simulink model "Exo_Origianl"  (R2023b)
settings: Solver=ode5  StartTime=0.0  StopTime=inf  FixedStep=dt  RelTol=1e-3  EnableMultiTasking=on
values from neighbouring files (symbols this model uses):
  A_0_a = 4.011    [Operator.m]
  A_0_h = 40.69    [Operator.m]
  A_0_k = 25.7    [Operator.m]
  A_1_a = 5.292    [Operator.m]
  A_1_h = 23.22    [Operator.m]
  A_1_k = -3.827    [Operator.m]
  A_2_a = -8.582    [Operator.m]
  A_2_h = -4.487    [Operator.m]
  A_2_k = -8.543    [Operator.m]
  A_3_a = -0.4755    [Operator.m]
  A_3_h = 0.3995    [Operator.m]
  A_3_k = 1.913    [Operator.m]
  A_4_a = 1.688    [Operator.m]
  A_4_k = 1.087    [Operator.m]
  A_5_a = -0.03504    [Operator.m]
  A_5_k = 2.054    [Operator.m]
  A_6_a = 1.298    [Operator.m]
  A_6_k = -0.3061    [Operator.m]
  amplitude = 0.8    [Operator.m]
  ankleStrategyInterval = 1.5    [Operator.m]
  B_1_a = 3.613    [Operator.m]
  B_1_h = -8.65    [Operator.m]
  B_1_k = -19.28    [Operator.m]
  B_2_a = -5.954    [Operator.m]
  B_2_h = 3.338    [Operator.m]
  B_2_k = 17.93    [Operator.m]
  B_3_a = 5.918    [Operator.m]
  B_3_h = 1.389    [Operator.m]
  B_3_k = 3.772    [Operator.m]
  B_4_a = -2.118    [Operator.m]
  B_4_k = 1.504    [Operator.m]
  B_5_a = 1.023    [Operator.m]
  B_5_k = 0.5838    [Operator.m]
  B_6_a = -0.7245    [Operator.m]
  B_6_k = -0.8958    [Operator.m]
  DCM_filter = 1 - dt/(dt+RC)    (= 0.926612305411)    [Operator.m]
  dt = 0.01    [Operator.m]
  frequency = 1.2    [Operator.m]
  gamma = fzero(eqn, 0.1)    [Operator.m]
  hipOffset = -17    [Operator.m]
  K_high = 0.5    [Operator.m]
  K_low = 0.5    [Operator.m]
  KD = 0.39    [Operator.m]
  Kp = 10    [Operator.m]
  l3 = userHeight*0.232    (= 15.776)    [Operator.m]
  l4 = userHeight*0.247    (= 16.796)    [Operator.m]
  l_c2 = ((0.29*34.66+0.63*6.07)/(6.07+34.66))/(0.52+0.19)*l2    (= 15.0425832454)    [Operator.m]
  l_c3 = 0.17/0.40*l3    (= 6.7048)    [Operator.m]
  l_c4 = ((0.19*3.52+0.43*1.05)/(3.52+1.05))/0.43*l4    (= 9.57536959951)    [Operator.m]
  l_foot = 11.25    [Operator.m]
  m2 = m2 + 2.2048*7.591    (= 119.8566368)    [Operator.m]
  m3 = m3 + 2.2048*1.715    (= 19.781232)    [Operator.m]
  m4 = userWeight*(0.0459+0.0169)    (= 10.048)    [Operator.m]
  m_Exo = 2.2048*1.647    (= 3.6313056)    [Operator.m]
  m_f = userWeight*0.0169    (= 2.704)    [Operator.m]
  maxTorque = 35    [Operator.m]
  P_t_ZMP_gain_Ankle = 0    [Operator.m]
  P_t_ZMP_gain_Hip = 0    [Operator.m]
  Phase_Left = 2+pi    (= 5.14159265359)    [Operator.m]
  Phase_Right = 2    [Operator.m]
  ramp = 2    [Operator.m]
  Strategy_filter = DCM_filter    (= 0.926612305411)    [Operator.m]
  strategySaturation = 10    [Operator.m]
  userHeight = 68    [Operator.m]
  userWeight = 160    [Operator.m]
undefined symbols (not defined in the file or in its folder): CAN_Device, DCMErrorPenalty, PEAK, Phase_Left_Knee_0, System, totalPowerPenalty
libraries: sldrtlib x35, simulink x16, rllib x1
(part 1 of 4)
settings Model: SimulationMode=external  ExtModeTrigDuration=60001  Creator=517541  LastModifiedBy=tschmidt
settings SolverCC: AlgebraicLoopSolver=TrustRegion
settings DataIOCC: ReturnWorkspaceOutputs=off
settings DebuggingCC: SolverPrmCheckMsg=warning  UnconnectedInputMsg=warning  UnconnectedOutputMsg=warning  UnconnectedLineMsg=warning  PregeneratedLibrarySubsystemCodeDiagnostic=none  SFUnexpectedBacktrackingDiag=warning  SFNoUnconditionalDefaultTransitionDiag=warning  SFExecutionAtInitializationDiag=none  ArithmeticOperatorsInVariantConditions=warning
settings HardwareCC: ProdBitPerLong=64  ProdHWDeviceType=Intel->x86-64 (Linux 64)
settings ModelReferenceCC: EnableRefExpFcnMdlSchedulingChecks=on  PropagateSignalLabelsOutOfModel=off
settings SFSimCC: SimUseLocalCustomCode=off  CustomCodeUndefinedFunction=UseInterfaceOnly
settings RTWCC: Description=Simulink Desktop Real-Time  SystemTargetFile=sldrt.tlc  TemplateMakefile=sldrt.tmf  RTWUseLocalCustomCode=off  RTWCompilerOptimization=on  DLArmComputeVersion=19.05
settings CodeAppCC: MaxIdLength=95  StateflowObjectComments=on
settings SimulinkDesktopRealTimeCC: TargetLibSuffix=_sldrt.a  TargetPreCompLibLocation=C:\Program Files\MATLAB\R2023b\toolbox\sldrt\lib\win64

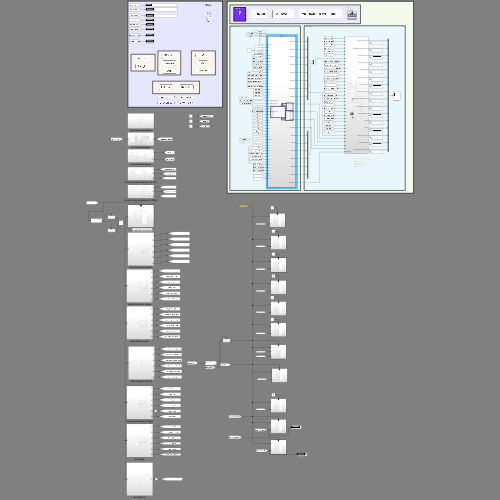
[thumbnail: Simulink's stored preview of the top-level diagram]
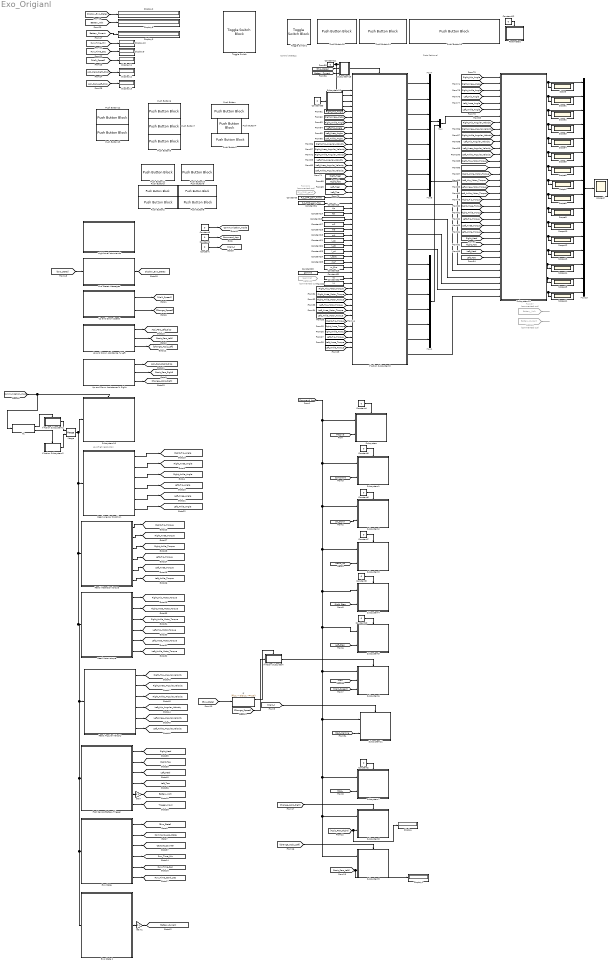
== system Exo_Origianl ==
  note: Control Strategy
  note: Data Retrieval
  note: Low/High resolution
  Constant{,1..2,4..12,33} (13 alike) : Constant  Value=0
  Constant13 : Constant  Value=Kp
  Constant14 : Constant  Value=KD
  Constant15 : Constant  Value=ankleStrategyInterval
  Constant17 : Constant  Value=m2
  Constant18 : Constant  Value=m3
  Constant19 : Constant  Value=m4
  Constant21 : Constant  Value=l_c2
  Constant22 : Constant  Value=l_c3
  Constant23 : Constant  Value=l_c4
  Constant24 : Constant  Value=l_foot
  Constant25 : Constant  Value=m_f
  Constant26 : Constant  Value=m_Exo
  Constant28 : Constant  Value=gamma
  Constant3 : Constant  Value=P_t_ZMP_gain_Ankle
  Constant31 : Constant  Value=l3
  Constant32 : Constant  Value=l4
  Constant34 : Constant  Value=P_t_ZMP_gain_Hip
  Display{,1..3,8..13} (10 alike) : Display
  Exo State : Subsystem
  Exo State 2 : Subsystem
  Exo States Messages : Subsystem
  Foot Sensor/Battery/Trigger : Subsystem
  From101 : From  Commented=on  GotoTag=P_t_ZMP_gain
  From102 : From  Commented=on  GotoTag=gamma
  From37 : From  Commented=on  GotoTag=Battery_Volt  TagVisibility=global
  From38 : From  Commented=on  GotoTag=Battery_Current  TagVisibility=global
  Gain : Gain  Gain=0.1
  Gain1 : Gain  Gain=0.1
  High-level commands : Subsystem
  If : If  IfExpression=(u1 > 0)&(u1 <= 10)
  If Action Subsystem : Subsystem  TreatAsAtomicUnit=on
  If Action Subsystem1 : Subsystem  TreatAsAtomicUnit=on
  If Action Subsystem2 : Subsystem  TreatAsAtomicUnit=on
  If Action Subsystem3 : Subsystem  TreatAsAtomicUnit=on
  If1 : If
  Merge : Merge
  Mux : Mux  Inputs=2
  Mux1 : Mux  Inputs=6
  Mux13 : Mux  Inputs=16
  Mux5 : Mux  Inputs=2
  Mux7 : Mux  Inputs=6
  Parameters : Subsystem
  Push Button : PushButtonBlock  ButtonText=Up Vel  OffValue=0.000000
  Push Button1 : PushButtonBlock  ButtonText=Down Vel
  Push Button10 : PushButtonBlock  ButtonText=Right_Step  OffValue=0.000000
  Push Button11 : PushButtonBlock  ButtonText=Left_Step  OffValue=0.000000
  Push Button12 : PushButtonBlock  ButtonText=Sit_Down  OffValue=0.000000
  Push Button13 : PushButtonBlock  ButtonText=Stand_Up  OffValue=0.000000
  Push Button14 : PushButtonBlock  ButtonText=Walk/Stop  ButtonType=Latch  OffValue=0.000000
  Push Button15 : PushButtonBlock  ButtonText=Acknowledge Parameters  OffValue=0.000000
  Push Button16 : PushButtonBlock  ButtonText=Activate  ButtonType=Latch  OffValue=0.000000
  Push Button2 : PushButtonBlock  ButtonText=Down Left %  OffValue=0.000000
  Push Button3 : PushButtonBlock  ButtonText=Up Left %  OffValue=0.000000
  Push Button4 : PushButtonBlock  ButtonText=Walk  OffValue=0.000000
  Push Button5 : PushButtonBlock  ButtonText=Stop  OffValue=0.000000
  Push Button6 : PushButtonBlock  ButtonText=Release  OffValue=0.000000
  Push Button7 : PushButtonBlock  ButtonText=Transparent  OffValue=0.000000
  Push Button8 : PushButtonBlock  ButtonText=Down Right %  OffValue=0.000000
  Push Button9 : PushButtonBlock  ButtonText=Up Right %  OffValue=0.000000
  Read Angular Possition : Subsystem
  Read Angular Velocity : Subsystem
  Read Interaction torque : Subsystem
  Read Motor torque : Subsystem
  Scope{,1..15} (16 alike) : Scope
  Subsystem : Subsystem
  Subsystem1 : Subsystem
  Subsystem10 : Subsystem
  Subsystem11 : Subsystem
  Subsystem12 : Subsystem
  Subsystem13 : Subsystem
  Subsystem15 : Subsystem
  Subsystem2 : Subsystem
  Subsystem3 : Subsystem
  Subsystem4 : Subsystem
  Subsystem5 : Subsystem
  Subsystem6 : Subsystem
  Subsystem7 : Subsystem
  Subsystem8 : Subsystem
  Subsystem9 : Subsystem
  Toggle Switch : ToggleSwitchBlock
      settings: Values={{'CAN', 'Bluetooth'}, [0 1]}
  Toggle Switch1 : ToggleSwitchBlock  LabelPosition=Hide
      settings: Values={{'Low resolution', 'High resolution'}, [1 0]}
  Up and Down Assistance % Left : Subsystem
  Up and Down Assistance % Right : Subsystem
  Up and Down Speed : Subsystem
  scopeAll : Scope
  tag scope: Assi_Perc_Left_Disp=global, Assi_Perc_Right_Disp=global, Battery_Current=global, Battery_Volt=global, Capture_Counter=global, Change_Assis_Right=global, Command_App=global, Command_App_State=global, Communication_mode=global, Display_Exo_States=global, Left_Ankle_Angle=global, Left_Ankle_Angular_Velocity=global, Left_Ankle_Motor_Torque=global, Left_Ankle_Torque=global, Left_Heel=global, Left_Hip_Angle=global, Left_Hip_Angular_Velocity=global, Left_Hip_Motor_Torque=global, Left_Hip_Torque=global, Left_Knee_Angle=global, Left_Knee_Angular_Velocity=global, Left_Knee_Motor_Torque=global, Left_Knee_Torque=global, Left_Toe=global, Right_Ankle_Angle=global, Right_Ankle_Angular_Velocity=global, Right_Ankle_Motor_Torque=global, Right_Ankle_Torque=global, Right_Heel=global, Right_Hip_Angle=global, Right_Hip_Angular_Velocity=global, Right_Hip_Motor_Torque=global, Right_Hip_Torque=global, Right_Knee_Angle=global, Right_Knee_Angular_Velocity=global, Right_Knee_Motor_Torque=global, Right_Knee_Torque=global, Right_Toe=global, Run_Time_Centi_Sec=global, Run_Time_Min=global, Run_Time_Sec=global, Trigger_Input=global
  wires:
  Constant1/1 -> [Command_App]
  [Compliant] -> Subsystem1/2(In2)
  Up and Down Speed/1(Out1) -> [Walk_Speed]
  [Sit_Down] -> Subsystem2/2(In2)
  [Stand_Up] -> Subsystem3/2(In2)
  [Right_Step] -> Subsystem4/2(In2)
  [Left_Step] -> Subsystem5/2(In2)
  [Passive] -> Subsystem/2(In2)
  Constant/1 -> [Walk_]
  Constant4/1 -> Subsystem/Trigger
  Constant10/1 -> Subsystem5/Trigger
  Constant8/1 -> Subsystem4/Trigger
  Constant7/1 -> Subsystem3/Trigger
  Constant6/1 -> Subsystem2/Trigger
  Constant5/1 -> Subsystem1/Trigger
  Up and Down Assistance % Right/3(Out3) -> [Change_Assis_Right]
  Up and Down Assistance % Right/2(Out2) -> [Assis_Perc_Right]
  Up and Down Assistance % Right/1(Out1) -> [Assi_Perc_Right_Disp]
  [Exo_State] -> Exo States Messages/1(In1)
  Exo States Messages/1(Out1) -> [Display_Exo_States]
  [Assi_Perc_Right_Disp] -> Display12/1
  [Assi_Perc_Left_Disp] -> Display13/1
  [Run_Time_Min] -> Display10/1
  [Display_Exo_States] -> Display2/1
  [Run_Time_Sec] -> Display9/1
  [Walk_Speed] -> Display11/1
  [Battery_Volt] -> Display8/1
  Read Interaction torque/4(Out4) -> [Left_Hip_Torque]
  Read Interaction torque/2(Out2) -> [Right_Knee_Torque]
  Read Interaction torque/3(Out3) -> [Right_Ankle_Torque]
  Read Interaction torque/6(Out6) -> [Left_Ankle_Torque]
  Read Interaction torque/1(Out1) -> [Right_Hip_Torque]
  Read Interaction torque/5(Out5) -> [Left_Knee_Torque]
  Read Motor torque/2(Out2) -> [Right_Knee_Motor_Torque]
  Read Motor torque/5(Out5) -> [Left_Knee_Motor_Torque]
  Read Motor torque/3(Out3) -> [Right_Ankle_Motor_Torque]
  Read Motor torque/1(Out1) -> [Right_Hip_Motor_Torque]
  Read Motor torque/6(Out6) -> [Left_Ankle_Motor_Torque]
  Read Motor torque/4(Out4) -> [Left_Hip_Motor_Torque]
  Foot Sensor/Battery/Trigger/4(Out4) -> [Left_Toe]
  Foot Sensor/Battery/Trigger/6(Out6) -> [Trigger_Input]
  Foot Sensor/Battery/Trigger/2(Out2) -> [Right_Toe]
  Foot Sensor/Battery/Trigger/1(Out1) -> [Right_Heel]
  Foot Sensor/Battery/Trigger/3(Out3) -> [Left_Heel]
  Exo State/4(Out4) -> [Run_Time_Min]
  Exo State/1(Out1) -> [Exo_State]
  Exo State/2(Out2) -> [Command_App_State]
  Exo State/5(Out5) -> [Run_Time_Sec]
  Exo State/6(Out6) -> [Run_Time_Centi_Sec]
  Exo State/3(Out3) -> [Capture_Counter]
  Gain/1 -> [Battery_Volt]
  Foot Sensor/Battery/Trigger/5(Out5) -> Gain/1
  Up and Down Assistance % Left/1(Out1) -> [Assi_Perc_Left_Disp]
  Up and Down Assistance % Left/2(Out2) -> [Assis_Perc_Left]
  Up and Down Assistance % Left/3(Out3) -> [Change_Assis_Left]
  [Start_Walking] -> Subsystem11/2(In2)
  [Assis_Perc_Right] -> Display/1, Subsystem8/2(In2)
  If/1 -> If Action Subsystem/Action
  [Assis_Perc_Left] -> Display1/1, Subsystem9/2(In2)
  [Stop_] -> Subsystem7/2(In2)
  [Change_Assis_Left] -> Subsystem9/Trigger
  [Change_Speed] -> If Action Subsystem/1(In1)
  [Walk_] -> Subsystem11/Trigger
  [Change_Assis_Right] -> Subsystem8/Trigger
  [Command_App] -> Subsystem/1(In1), Subsystem1/1(In1), Subsystem2/1(In1), Subsystem3/1(In1), Subsystem4/1(In1), Subsystem11/1(In1), Subsystem9/1(In1), Subsystem8/1(In1), Subsystem7/1(In1), Subsystem6/1(In1), Subsystem5/1(In1)
  [Walk] -> Subsystem6/2(In2)
  If Action Subsystem/1(Out1) -> Subsystem6/Trigger
  Constant2/1 -> Subsystem7/Trigger
  [Walk_Speed] -> Subsystem6/3(In3)
  [Exo_State] -> If/1
  Up and Down Speed/2(Out2) -> [Change_Speed]
  [Communication_mode] -> If1/1, Subsystem10/Trigger
  Constant9/1 -> [Communication_mode]
  Read Angular Possition/1(Out1) -> [Right_Hip_Angle]
  Read Angular Possition/2(Out2) -> [Right_Knee_Angle]
  Read Angular Possition/3(Out3) -> [Right_Ankle_Angle]
  Read Angular Possition/4(Out4) -> [Left_Hip_Angle]
  Read Angular Possition/5(Out5) -> [Left_Knee_Angle]
  Read Angular Possition/6(Out6) -> [Left_Ankle_Angle]
  If1/1 -> If Action Subsystem1/Action
  If Action Subsystem1/1(Out1) -> Merge/1
  If1/2 -> If Action Subsystem2/Action
  If Action Subsystem2/1(Out1) -> Merge/2
  Merge/1 -> Read Angular Velocity/1(Input), Exo State 2/1(Input), Exo State/1(Input), Foot Sensor/Battery/Trigger/1(Input), Read Motor torque/1(Input), Read Interaction torque/1(Input), Read Angular Possition/1(Input), Subsystem10/1(In1)
  Exo State 2/1(Out1) -> Gain1/1
  Gain1/1 -> [Battery_Current]
  [Battery_Current] -> Display3/1
  Read Angular Velocity/4(Out4) -> [Left_Hip_Angular_Velocity]
  Read Angular Velocity/6(Out6) -> [Left_Ankle_Angular_Velocity]
  Read Angular Velocity/3(Out3) -> [Right_Ankle_Angular_Velocity]
  Read Angular Velocity/5(Out5) -> [Left_Knee_Angular_Velocity]
  Read Angular Velocity/2(Out2) -> [Right_Knee_Angular_Velocity]
  Read Angular Velocity/1(Out1) -> [Right_Hip_Angular_Velocity]
  Constant11/1 -> If Action Subsystem3/1(Trigger), Subsystem15/1(Input)
  [Right_Hip_Angle] -> If Action Subsystem3/5(RHAA)
  [Right_Knee_Angle] -> If Action Subsystem3/6(RKAA)
  [Right_Ankle_Angle] -> If Action Subsystem3/7(RAAA)
  [Left_Hip_Angle] -> If Action Subsystem3/8(LHAA)
  [Left_Knee_Angle] -> If Action Subsystem3/9(LKAA)
  [Left_Ankle_Angle] -> If Action Subsystem3/10(LAAA)
  [Right_Heel] -> If Action Subsystem3/17(RHP)
  [Right_Toe] -> If Action Subsystem3/18(RTP)
  [Left_Heel] -> If Action Subsystem3/19(LHP)
  [Left_Toe] -> If Action Subsystem3/20(LTP)
  [Left_Ankle_Angular_Velocity] -> If Action Subsystem3/16(Input5)
  [Right_Ankle_Angular_Velocity] -> If Action Subsystem3/13(Input4)
  Subsystem15/1(Trigger) -> If Action Subsystem3/Action
  [Right_Hip_Angular_Velocity] -> If Action Subsystem3/11(Input2)
  [Left_Hip_Angular_Velocity] -> If Action Subsystem3/14(Input14)
  [Left_Knee_Angular_Velocity] -> If Action Subsystem3/15(Input15)
  [Right_Knee_Angular_Velocity] -> If Action Subsystem3/12(Input3)
  Constant12/1 -> Parameters/Trigger
  Subsystem12/1(amplitude) -> If Action Subsystem3/2(Input6)
  Subsystem12/2(frequency) -> If Action Subsystem3/3(Input7)
  Subsystem12/3(hipOffset) -> If Action Subsystem3/4(Input8)
  If Action Subsystem3/6(LAA Desired) -> Mux7/6
  If Action Subsystem3/5(LKA Desired) -> Mux7/5
  If Action Subsystem3/4(LHA Desired) -> Mux7/4
  If Action Subsystem3/3(RAA Desired) -> Mux7/3
  If Action Subsystem3/2(RKA Desired) -> Mux7/2
  If Action Subsystem3/1(RHA Desired) -> Mux7/1
  If Action Subsystem3/7(Right Strategy) -> Mux5/1
  If Action Subsystem3/8(Left Strategy) -> Mux5/2
  Constant13/1 -> If Action Subsystem3/23(Kp)
  Constant14/1 -> If Action Subsystem3/24(KD)
  Constant15/1 -> If Action Subsystem3/25(ankleStrategyInterval)
  Constant17/1 -> If Action Subsystem3/26(m2)
  Constant18/1 -> If Action Subsystem3/27(m3)
  Constant19/1 -> If Action Subsystem3/28(m4)
  Constant21/1 -> If Action Subsystem3/29(l_c2)
  Constant22/1 -> If Action Subsystem3/30(l_c3)
  Constant23/1 -> If Action Subsystem3/31(l_c4)
  Constant24/1 -> If Action Subsystem3/32(I1)
  Constant25/1 -> If Action Subsystem3/33(I2)
  Constant26/1 -> If Action Subsystem3/34(I3)
  Constant3/1 -> If Action Subsystem3/21(P_t_ZMP_Gain_Ankle)
  Constant28/1 -> If Action Subsystem3/35(gamma)
  Constant32/1 -> If Action Subsystem3/37(l4)
  Constant31/1 -> If Action Subsystem3/36(l3)
  Constant33/1 -> Subsystem12/1(Input)
  [Exo_State] -> Subsystem15/2(Input1)
  Mux13/1 -> scopeAll/1
  If Action Subsystem3/9(Ankle) -> Subsystem13/31(31)
  [Right_Hip_Angle] -> Subsystem13/1(In1)
  [Right_Knee_Angle] -> Subsystem13/2(In2)
  [Right_Ankle_Angle] -> Subsystem13/3(In3)
  [Left_Hip_Angle] -> Subsystem13/4(In4)
  [Left_Knee_Angle] -> Subsystem13/5(In5)
  [Left_Ankle_Angle] -> Subsystem13/6(In6)
  [Right_Hip_Angular_Velocity] -> Subsystem13/8(In7)
  [Right_Knee_Angular_Velocity] -> Subsystem13/9(In8)
  [Right_Ankle_Angular_Velocity] -> Subsystem13/10(In9)
  [Left_Hip_Angular_Velocity] -> Subsystem13/11(In10)
  [Left_Knee_Angular_Velocity] -> Subsystem13/12(In11)
  [Left_Ankle_Angular_Velocity] -> Subsystem13/13(In12)
  [Right_Heel] -> Subsystem13/26(In13)
  [Right_Toe] -> Subsystem13/27(In14)
  [Left_Heel] -> Subsystem13/28(In15)
  [Left_Toe] -> Subsystem13/29(In16)
  [Right_Hip_Motor_Torque] -> Subsystem13/14(In17)
  [Right_Knee_Motor_Torque] -> Subsystem13/15(In18)
  [Right_Ankle_Motor_Torque] -> Subsystem13/16(In19)
  [Left_Hip_Motor_Torque] -> Subsystem13/17(In20)
  [Left_Knee_Motor_Torque] -> Subsystem13/18(In21)
  [Left_Ankle_Motor_Torque] -> Subsystem13/19(In22)
  [Right_Hip_Torque] -> Subsystem13/20(In23)
  [Right_Knee_Torque] -> Subsystem13/21(In24)
  [Right_Ankle_Torque] -> Subsystem13/22(In26)
  [Left_Hip_Torque] -> Subsystem13/23(In27)
  [Left_Knee_Torque] -> Subsystem13/24(In28)
  [Left_Ankle_Torque] -> Subsystem13/25(In30)
  Mux7/1 -> Mux/1
  Mux5/1 -> Subsystem13/30(In29)
  Subsystem13/1(Actual Joint Angles (1-6)) -> Mux13/1, Scope/1
  Subsystem13/2(Desired/Initial Joint Angles (7-18)) -> Scope1/1, Mux13/2
  Subsystem13/3(Joint Velocities (19-24)) -> Scope2/1, Mux13/3
  Subsystem13/4(Motor Torque (24-30)) -> Scope3/1, Mux13/4
  Subsystem13/5(HRI Torque (31-36)) -> Scope4/1, Mux13/5
  Subsystem13/6(Foot Pressure (37-40)) -> Scope5/1, Mux13/6
  Subsystem13/7(Joint Power (41-46)) -> Mux13/7, Scope6/1
  Subsystem13/8(Strategy Torque (41-43)) -> Scope7/1, Mux13/8
  Subsystem13/9("Desired Torques, DCM Error (44-50)") -> Scope8/1, Mux13/9
  Subsystem13/14(Ankle Strategy (75-77)) -> Scope14/1, Mux13/14
  Subsystem13/13(KD (74)) -> Mux13/13, Scope13/1
  Subsystem13/12(Kp (73)) -> Scope12/1, Mux13/12
  Subsystem13/16(Reinforcement Learning (84-86)) -> Mux13/16, Scope11/1
  Subsystem13/11(DCM Strategy (53-72)) -> Scope10/1, Mux13/11
  Subsystem13/10(Current Step/Time (51-52)) -> Scope9/1, Mux13/10
  If Action Subsystem3/10(currentStep/Time) -> Subsystem13/32(32)
  If Action Subsystem3/11(Ankle Strategy) -> Subsystem13/33(Input)
  Subsystem13/15(Parameters (78-83)) -> Scope15/1, Mux13/15
  [Right_Hip_Motor_Torque] -> If Action Subsystem3/38(Input1)
  [Right_Knee_Motor_Torque] -> If Action Subsystem3/39(Input9)
  [Right_Ankle_Motor_Torque] -> If Action Subsystem3/40(Input10)
  [Left_Hip_Motor_Torque] -> If Action Subsystem3/41(Input11)
  [Left_Knee_Motor_Torque] -> If Action Subsystem3/42(Input12)
  [Left_Ankle_Motor_Torque] -> If Action Subsystem3/43(Input13)
  Constant34/1 -> If Action Subsystem3/22(P_t_ZMP_Gain_hip)
  If Action Subsystem3/12(Hip Strategy) -> Subsystem13/34(34)
  [Battery_Current] -> Subsystem15/3(Input2)
  [Right_Hip_Torque] -> If Action Subsystem3/44(Input16)
  [Right_Knee_Torque] -> If Action Subsystem3/45(Input17)
  [Right_Ankle_Torque] -> If Action Subsystem3/46(Input18)
  [Left_Hip_Torque] -> If Action Subsystem3/47(Input19)
  [Left_Knee_Torque] -> If Action Subsystem3/48(Input31)
  [Left_Ankle_Torque] -> If Action Subsystem3/49(Input32)
  If Action Subsystem3/13(LAA Initial) -> Mux1/1
  If Action Subsystem3/14(LKA Initial) -> Mux1/2
  If Action Subsystem3/15(LHA Initial) -> Mux1/3
  If Action Subsystem3/16(RAA Initial) -> Mux1/4
  If Action Subsystem3/17(RKA Initial) -> Mux1/5
  If Action Subsystem3/18(RHA Initial) -> Mux1/6
  Mux/1 -> Subsystem13/7(In25)
  Mux1/1 -> Mux/2
  If Action Subsystem3/19(Strategy Gain) -> Subsystem13/35(Strategy Gain)
  From38/1 -> ?
  From37/1 -> ?

== system Exo_Origianl/Exo State ==
  Input : Inport
  If : If  IfExpression=u1 == 1
  If Action Subsystem : Subsystem  TreatAsAtomicUnit=on
  If Action Subsystem1 : Subsystem  TreatAsAtomicUnit=on
  Merge{,1..5} (6 alike) : Merge
  Out1 : Outport
  Out2 : Outport  Port=2
  Out3 : Outport  Port=3
  Out4 : Outport  Port=4
  Out5 : Outport  Port=5
  Out6 : Outport  Port=6
  wires:
  Input/1 -> If/1
  Merge/1 -> Out1/1
  If Action Subsystem/1(Out7) -> Merge/1
  If/1 -> If Action Subsystem/Action
  If/2 -> If Action Subsystem1/Action
  Merge1/1 -> Out2/1
  Merge2/1 -> Out3/1
  Merge3/1 -> Out4/1
  Merge4/1 -> Out5/1
  Merge5/1 -> Out6/1
  If Action Subsystem/2(Out8) -> Merge1/1
  If Action Subsystem/3(Out9) -> Merge2/1
  If Action Subsystem/4(Out10) -> Merge3/1
  If Action Subsystem/5(Out11) -> Merge4/1
  If Action Subsystem/6(Out12) -> Merge5/1
  If Action Subsystem1/1(Out1) -> Merge/2
  If Action Subsystem1/2(Out2) -> Merge1/2
  If Action Subsystem1/3(Out3) -> Merge2/2
  If Action Subsystem1/4(Out4) -> Merge3/2
  If Action Subsystem1/5(Out5) -> Merge4/2
  If Action Subsystem1/6(Out6) -> Merge5/2

== system Exo_Origianl/Exo State 2 ==
  Input : Inport
  If : If  IfExpression=u1 == 1
  If Action Subsystem : Subsystem  TreatAsAtomicUnit=on
  If Action Subsystem1 : Subsystem  TreatAsAtomicUnit=on
  Merge : Merge
  Out1 : Outport
  wires:
  Input/1 -> If/1
  Merge/1 -> Out1/1
  If Action Subsystem/1(Out7) -> Merge/1
  If/1 -> If Action Subsystem/Action
  If/2 -> If Action Subsystem1/Action
  If Action Subsystem1/1(Out1) -> Merge/2

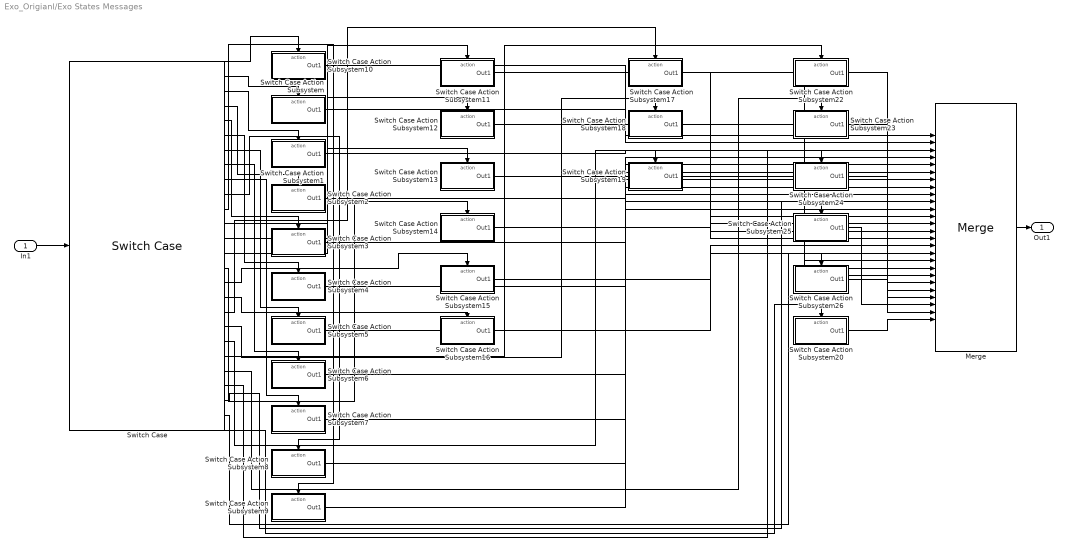
== system Exo_Origianl/Exo States Messages ==
  In1 : Inport
  Merge : Merge  Inputs=26
  Switch Case : SwitchCase  CaseConditions={0,1,2,3,4,5,6,7,8,9,10,11,12,13,14,15,16,17,18,19,21,22,23,24,25,26}  ShowDefaultCase=off
  Switch Case Action Subsystem : Subsystem  TreatAsAtomicUnit=on
  Switch Case Action Subsystem1 : Subsystem  TreatAsAtomicUnit=on
  Switch Case Action Subsystem10 : Subsystem  TreatAsAtomicUnit=on
  Switch Case Action Subsystem11 : Subsystem  TreatAsAtomicUnit=on
  Switch Case Action Subsystem12 : Subsystem  TreatAsAtomicUnit=on
  Switch Case Action Subsystem13 : Subsystem  TreatAsAtomicUnit=on
  Switch Case Action Subsystem14 : Subsystem  TreatAsAtomicUnit=on
  Switch Case Action Subsystem15 : Subsystem  TreatAsAtomicUnit=on
  Switch Case Action Subsystem16 : Subsystem  TreatAsAtomicUnit=on
  Switch Case Action Subsystem17 : Subsystem  TreatAsAtomicUnit=on
  Switch Case Action Subsystem18 : Subsystem  TreatAsAtomicUnit=on
  Switch Case Action Subsystem19 : Subsystem  TreatAsAtomicUnit=on
  Switch Case Action Subsystem2 : Subsystem  TreatAsAtomicUnit=on
  Switch Case Action Subsystem20 : Subsystem  TreatAsAtomicUnit=on
  Switch Case Action Subsystem22 : Subsystem  TreatAsAtomicUnit=on
  Switch Case Action Subsystem23 : Subsystem  TreatAsAtomicUnit=on
  Switch Case Action Subsystem24 : Subsystem  TreatAsAtomicUnit=on
  Switch Case Action Subsystem25 : Subsystem  TreatAsAtomicUnit=on
  Switch Case Action Subsystem26 : Subsystem  TreatAsAtomicUnit=on
  Switch Case Action Subsystem3 : Subsystem  TreatAsAtomicUnit=on
  Switch Case Action Subsystem4 : Subsystem  TreatAsAtomicUnit=on
  Switch Case Action Subsystem5 : Subsystem  TreatAsAtomicUnit=on
  Switch Case Action Subsystem6 : Subsystem  TreatAsAtomicUnit=on
  Switch Case Action Subsystem7 : Subsystem  TreatAsAtomicUnit=on
  Switch Case Action Subsystem8 : Subsystem  TreatAsAtomicUnit=on
  Switch Case Action Subsystem9 : Subsystem  TreatAsAtomicUnit=on
  Out1 : Outport
  wires:
  Switch Case/2 -> Switch Case Action Subsystem/Action
  Switch Case/3 -> Switch Case Action Subsystem1/Action
  Switch Case/4 -> Switch Case Action Subsystem2/Action
  Switch Case/5 -> Switch Case Action Subsystem3/Action
  Switch Case/6 -> Switch Case Action Subsystem4/Action
  Switch Case/7 -> Switch Case Action Subsystem5/Action
  Switch Case/8 -> Switch Case Action Subsystem6/Action
  Switch Case/9 -> Switch Case Action Subsystem7/Action
  Switch Case/10 -> Switch Case Action Subsystem8/Action
  Switch Case/11 -> Switch Case Action Subsystem9/Action
  Switch Case/1 -> Switch Case Action Subsystem10/Action
  Switch Case/12 -> Switch Case Action Subsystem11/Action
  Switch Case/13 -> Switch Case Action Subsystem12/Action
  Switch Case/14 -> Switch Case Action Subsystem13/Action
  Switch Case/15 -> Switch Case Action Subsystem14/Action
  Switch Case/16 -> Switch Case Action Subsystem15/Action
  Switch Case/17 -> Switch Case Action Subsystem16/Action
  Switch Case/18 -> Switch Case Action Subsystem17/Action
  Switch Case/19 -> Switch Case Action Subsystem18/Action
  Switch Case/20 -> Switch Case Action Subsystem19/Action
  In1/1 -> Switch Case/1
  Switch Case/21 -> Switch Case Action Subsystem22/Action
  Switch Case/22 -> Switch Case Action Subsystem23/Action
  Switch Case/23 -> Switch Case Action Subsystem24/Action
  Switch Case/24 -> Switch Case Action Subsystem25/Action
  Switch Case/25 -> Switch Case Action Subsystem26/Action
  Switch Case/26 -> Switch Case Action Subsystem20/Action
  Switch Case Action Subsystem10/1(Out1) -> Merge/1
  Switch Case Action Subsystem/1(Out1) -> Merge/2
  Switch Case Action Subsystem1/1(Out1) -> Merge/3
  Switch Case Action Subsystem2/1(Out1) -> Merge/4
  Switch Case Action Subsystem3/1(Out1) -> Merge/5
  Switch Case Action Subsystem4/1(Out1) -> Merge/6
  Switch Case Action Subsystem5/1(Out1) -> Merge/7
  Switch Case Action Subsystem6/1(Out1) -> Merge/8
  Switch Case Action Subsystem7/1(Out1) -> Merge/9
  Switch Case Action Subsystem8/1(Out1) -> Merge/10
  Switch Case Action Subsystem9/1(Out1) -> Merge/11
  Switch Case Action Subsystem11/1(Out1) -> Merge/12
  Switch Case Action Subsystem12/1(Out1) -> Merge/13
  Switch Case Action Subsystem13/1(Out1) -> Merge/14
  Switch Case Action Subsystem14/1(Out1) -> Merge/15
  Switch Case Action Subsystem15/1(Out1) -> Merge/16
  Switch Case Action Subsystem16/1(Out1) -> Merge/17
  Switch Case Action Subsystem17/1(Out1) -> Merge/18
  Switch Case Action Subsystem18/1(Out1) -> Merge/19
  Switch Case Action Subsystem19/1(Out1) -> Merge/20
  Switch Case Action Subsystem22/1(Out1) -> Merge/21
  Switch Case Action Subsystem23/1(Out1) -> Merge/22
  Switch Case Action Subsystem24/1(Out1) -> Merge/23
  Switch Case Action Subsystem25/1(Out1) -> Merge/24
  Switch Case Action Subsystem26/1(Out1) -> Merge/25
  Switch Case Action Subsystem20/1(Out1) -> Merge/26
  Merge/1 -> Out1/1

== system Exo_Origianl/Foot Sensor//Battery//Trigger ==
  Input : Inport
  If : If  IfExpression=u1 == 1
  If Action Subsystem : Subsystem  TreatAsAtomicUnit=on
  If Action Subsystem1 : Subsystem  TreatAsAtomicUnit=on
  Merge{,1..5} (6 alike) : Merge
  Out1 : Outport
  Out2 : Outport  Port=2
  Out3 : Outport  Port=3
  Out4 : Outport  Port=4
  Out5 : Outport  Port=5
  Out6 : Outport  Port=6
  wires:
  Input/1 -> If/1
  Merge/1 -> Out1/1
  If Action Subsystem/1(Out7) -> Merge/1
  If/1 -> If Action Subsystem/Action
  If/2 -> If Action Subsystem1/Action
  Merge1/1 -> Out2/1
  Merge2/1 -> Out3/1
  Merge3/1 -> Out4/1
  Merge4/1 -> Out5/1
  Merge5/1 -> Out6/1
  If Action Subsystem/2(Out8) -> Merge1/1
  If Action Subsystem/3(Out9) -> Merge2/1
  If Action Subsystem/4(Out10) -> Merge3/1
  If Action Subsystem/5(Out11) -> Merge4/1
  If Action Subsystem/6(Out12) -> Merge5/1
  If Action Subsystem1/1(Out1) -> Merge/2
  If Action Subsystem1/2(Out2) -> Merge1/2
  If Action Subsystem1/3(Out3) -> Merge2/2
  If Action Subsystem1/4(Out4) -> Merge3/2
  If Action Subsystem1/5(Out5) -> Merge4/2
  If Action Subsystem1/6(Out6) -> Merge5/2

== system Exo_Origianl/High-level commands ==
  Constant : Constant  Value=0
  Constant1 : Constant  Value=11
  Constant2 : Constant  Value=12
  Constant3 : Constant  Value=23
  Constant4 : Constant  Value=24
  Constant5 : Constant  Value=21
  Constant6 : Constant  Value=22
  Constant7 : Constant  Value=10
  Constant8 : Constant
  tag scope: Compliant=global, Left_Step=global, Passive=global, Right_Step=global, Sit_Down=global, Stand_Up=global, Start_Walking=global, Stop_=global, Walk=global
  wires:
  Constant1/1 -> [Passive]
  Constant2/1 -> [Compliant]
  Constant/1 -> [Stop_]
  Constant3/1 -> [Right_Step]
  Constant4/1 -> [Left_Step]
  Constant5/1 -> [Stand_Up]
  Constant6/1 -> [Sit_Down]
  Constant7/1 -> [Walk]
  Constant8/1 -> [Start_Walking]

== system Exo_Origianl/If Action Subsystem ==
  In1 : Inport
  Action Port : ActionPort  ActionPortLabel=if((u1 > 0)&(u1 <= 10))
  Out1 : Outport
  wires:
  In1/1 -> Out1/1

== system Exo_Origianl/If Action Subsystem1 ==
  Action Port : ActionPort  ActionPortLabel=if(u1 > 0)
  Constant : Constant
  Out1 : Outport
  wires:
  Constant/1 -> Out1/1

== system Exo_Origianl/If Action Subsystem2 ==
  Action Port : ActionPort  ActionPortLabel=else
  Constant : Constant  Value=3
  Out1 : Outport
  wires:
  Constant/1 -> Out1/1

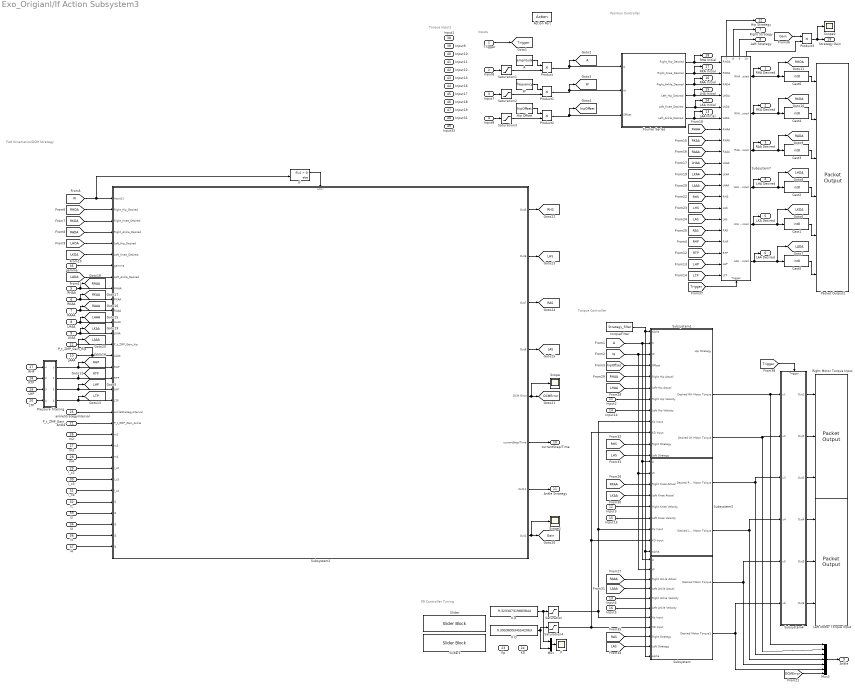
== system Exo_Origianl/If Action Subsystem3 ==
  note: Fwd Kinematics/DCM Strategy
  note: PD Controller Tuning
  note: Inputs
  note: Torque Controller
  note: Position Controller
  note: Torque Inputs
  Trigger : Inport
  Input6 : Inport  Port=2
  Input7 : Inport  Port=3
  Input8 : Inport  Port=4
  RHAA : Inport  Port=5
  RKAA : Inport  Port=6
  RAAA : Inport  Port=7
  LHAA : Inport  Port=8
  LKAA : Inport  Port=9
  LAAA : Inport  Port=10
  Input2 : Inport  Port=11
  Input3 : Inport  Port=12
  Input4 : Inport  Port=13
  Input14 : Inport  Port=14
  Input15 : Inport  Port=15
  Input5 : Inport  Port=16
  RHP : Inport  Port=17
  RTP : Inport  Port=18
  LHP : Inport  Port=19
  LTP : Inport  Port=20
  P_t_ZMP_Gain_Ankle : Inport  Port=21
  P_t_ZMP_Gain_hip : Inport  Port=22
  Kp : Inport  Port=23
  KD : Inport  Port=24
  ankleStrategyInterval : Inport  Port=25
  m2 : Inport  Port=26
  m3 : Inport  Port=27
  m4 : Inport  Port=28
  l_c2 : Inport  Port=29
  l_c3 : Inport  Port=30
  l_c4 : Inport  Port=31
  I1 : Inport  Port=32
  I2 : Inport  Port=33
  I3 : Inport  Port=34
  gamma : Inport  Port=35
  l3 : Inport  Port=36
  l4 : Inport  Port=37
  Input1 : Inport  Port=38
  Input9 : Inport  Port=39
  Input10 : Inport  Port=40
  Input11 : Inport  Port=41
  Input12 : Inport  Port=42
  Input13 : Inport  Port=43
  Input16 : Inport  Port=44
  Input17 : Inport  Port=45
  Input18 : Inport  Port=46
  Input19 : Inport  Port=47
  Input31 : Inport  Port=48
  Input32 : Inport  Port=49
  Action Port : ActionPort  ActionPortLabel=if(u1 > 0)
  A : Constant  Value=amplitude
  Cast{1..6} (6 alike) : DataTypeConversion  OutDataTypeStr=int8  SaturateOnIntegerOverflow=off  RndMeth=Floor
  Fourier Series : Subsystem
  From1 : From  TagVisibility=global
  Goto2 : Goto  TagVisibility=global
  Hip Offset : Constant  Value=hipOffset
  If : If
  K : Scope
  K D : Constant  Value=0.3959899345542063
  K p : Constant  Value=9.323307319883844
  Left Motor Torque Input : sldrtlib/Packet Output  SampleTime=-1  MaxMissedTicks=100  ShowMissedTicks=off  YieldWhenWaiting=off  DrvName=PEAK-System/CAN_Device  DrvAddress=81  DrvOptions=[0 0 0 0 1000 0 0 1 5 2 1 3 1]  PacketSize=6  DataTypes={'int16','int16','int16'}  ShowReady=off  ShowError=off  PacketID=2048e0 + (84)  ByteOrder=1  InitialValue=[]  FinalValue=[]
      settings: AttributesFormatString=PEAK-System\nCAN Device [81]
  Mux : Mux  Inputs=2
  Mux3 : Mux  Inputs=7
  Packet Output2 : sldrtlib/Packet Output  SampleTime=-1  MaxMissedTicks=100  ShowMissedTicks=off  YieldWhenWaiting=off  DrvName=PEAK-System/CAN_Device  DrvAddress=81  DrvOptions=[0 0 0 0 1000 0 0 1 5 2 1 3 1]  PacketSize=6  DataTypes={'int8','int8','int8','int8','int8','int8'}  ShowReady=off  ShowError=off  PacketID=2048e0 + (72)  ByteOrder=2  InitialValue=[]  FinalValue=[]
      settings: AttributesFormatString=PEAK-System\nCAN Device [81]
  Pressure filtering : Subsystem
  Product{,1..3} (4 alike) : Product
  Right Motor Torque Input : sldrtlib/Packet Output  SampleTime=-1  MaxMissedTicks=100  ShowMissedTicks=off  YieldWhenWaiting=off  DrvName=PEAK-System/CAN_Device  DrvAddress=81  DrvOptions=[0 0 0 0 1000 0 0 1 5 2 1 3 1]  PacketSize=6  DataTypes={'int16','int16','int16'}  ShowReady=off  ShowError=off  PacketID=2048e0 + (83)  ByteOrder=1  InitialValue=[]  FinalValue=[]
      settings: AttributesFormatString=PEAK-System\nCAN Device [81]
  Saturation : Saturate  UpperLimit=12  LowerLimit=0
  Saturation1 : Saturate  UpperLimit=1  LowerLimit=0
  Saturation2 : Saturate  UpperLimit=1  LowerLimit=0
  Saturation3 : Saturate  UpperLimit=1  LowerLimit=0
  Saturation4 : Saturate  UpperLimit=0.6  LowerLimit=0
  Scope : Scope
  Scope1 : Scope
  Scope2 : Scope
  Slider : SliderBlock  ScaleMax=12
  Slider1 : SliderBlock  ScaleMax=0.6
  Subsystem : Subsystem
  Subsystem1 : Subsystem
  Subsystem2 : Subsystem
  Subsystem3 : Subsystem
  Subsystem4 : Subsystem
      settings: PortSchema="{\"entries\":[{\"content\":{\"sides\":[{\"content\":{\"connectorIds\":[\"In1\",\"In2\",\"In3\",\"In4\",\"In5\",\"In6\"]},\"type\":\"ConnectorPlacement.EquallySpacedRectSide\",\"uuid\":\"ad775570-94cb-4a22-874c-8198f45043ae\"},{\"content\":{\"connectorIds\":[\"Out1\",\"Out2\",\"Out3\",\"Out4\",\"Out5\",\"Out6\"],\"side\":\"RIGHT\"},\"type\":\"ConnectorPlacement.EquallySpacedRectSide\",\"uuid\":\"c1dd8354-c582-4e42-877c-8f412df42689\"},{\"content\":{\"connectorIds\":[\"In7\"],\"side\":\"TOP\"},\"type\":\"ConnectorPlacement.EquallySpacedRectSide\",\"uuid\":\"911fbb41-8880-426f-9e94-7eaf95163f48\"}]},\"type\":\"ConnectorPlacement.EquallySpacedConnector\",\"uuid\":\"b831d7f8-8bd4-4758-8c6b-87675d565760\"}],\"packageUris\":[\"http://schema.mathworks.com/mf0/Connector/R2020b\"],\"version\":\"1.0\"}"
  Subsystem7 : Subsystem
      settings: PortSchema="{\"entries\":[{\"content\":{\"sides\":[{\"content\":{\"connectorIds\":[\"In1\",\"In2\",\"In3\",\"In4\",\"In5\",\"In6\",\"In7\",\"In8\",\"In9\",\"In10\",\"In11\",\"In12\",\"In13\",\"In14\",\"In15\",\"In16\",\"In17\",\"In18\",\"In19\",\"In20\"]},\"type\":\"ConnectorPlacement.EquallySpacedRectSide\",\"uuid\":\"1310c732-5ee3-486f-8410-0ef5c9f4f0a3\"},{\"content\":{\"connectorIds\":[\"Out1\",\"Out2\",\"Out3\",\"Out4\",\"Out5\",\"Out6\"],\"side\":\"RIGHT\"},\"type\":\"ConnectorPlacement.EquallySpacedRectSide\",\"uuid\":\"a3d0c36b-1fc5-4f72-9584-afe2fb03425e\"},{\"content\":{\"connectorIds\":[\"Out7\",\"Out8\",\"Out9\",\"Out10\"],\"side\":\"TOP\"},\"type\":\"ConnectorPlacement.EquallySpacedRectSide\",\"uuid\":\"2374624b-1290-4c4f-8ed5-af79ce858140\"},{\"content\":{\"connectorIds\":[\"In21\"],\"side\":\"BOTTOM\"},\"type\":\"ConnectorPlacement.EquallySpacedRectSide\",\"uuid\":\"5e7b8829-fa25-42f2-bc7d-9679c56e7627\"}]},\"type\":\"ConnectorPlacement.EquallySpacedConnector\",\"uuid\":\"1aa69e7d-787a-44aa-b8d3-106f13a75bb6\"}],\"packageUris\":[\"http://schema.mathworks.com/mf0/Connector/R2020b\"],\"version\":\"1.0\"}"
  W : Constant  Value=frequency
  torqueFilter : Constant  Value=Strategy_filter
  RHA Desired : Outport
  RKA Desired : Outport  Port=2
  RAA Desired : Outport  Port=3
  LHA Desired : Outport  Port=4
  LKA Desired : Outport  Port=5
  LAA Desired : Outport  Port=6
  Right Strategy : Outport  Port=7
  Left Strategy : Outport  Port=8
  Ankle : Outport  Port=9
  currentStep/Time : Outport  Port=10
  Ankle Strategy : Outport  Port=11
  Hip Strategy : Outport  Port=12
  LAA Initial : Outport  Port=13
  LKA Initial : Outport  Port=14
  LHA Initial : Outport  Port=15
  RAA Initial : Outport  Port=16
  RKA Initial : Outport  Port=17
  RHA Initial : Outport  Port=18
  Strategy Gain : Outport  Port=19
  tag scope: DCMError=global, Gain=global, LAAA=global, LADA=global, LAS=global, LHAA=global, LHDA=global, LHP=global, LHS=global, LKAA=global, LKDA=global, LTP=global, RAAA=global, RADA=global, RAS=global, RHAA=global, RHDA=global, RHP=global, RHS=global, RKAA=global, RKDA=global, RTP=global, Trigger=global, W=global, hipOffset=global
  wires:
  W/1 -> Product1/1
  Saturation1/1 -> Product/2
  Product/1 -> Goto2/1, Fourier Series/1(A)
  Input8/1 -> Saturation3/1
  A/1 -> Product/1
  Saturation3/1 -> Product2/2
  Product2/1 -> [hipOffset], Fourier Series/3(Offset)
  Saturation2/1 -> Product1/2
  Product1/1 -> [W], Fourier Series/2(W)
  Input6/1 -> Saturation1/1
  Hip Offset/1 -> Product2/1
  Input7/1 -> Saturation2/1
  Input4/1 -> Subsystem/5(Right Ankle Velocity)
  Input5/1 -> Subsystem/6(Left Ankle Velocity)
  Subsystem/1(Desired Motor Torque) -> Subsystem4/5(u5), Mux3/5
  Subsystem/2(Desired Motor Torque1) -> Mux3/6, Subsystem4/6(u6)
  Mux3/1 -> Ankle/1
  Input2/1 -> Subsystem1/7(Right Hip Velocity)
  Input14/1 -> Subsystem1/8(Left Hip Velocity)
  Input3/1 -> Subsystem3/5(Right Knee Velocity)
  Input15/1 -> Subsystem3/6(Left Knee Velocity)
  Subsystem1/2(Desired RH Motor Torque) -> Subsystem4/1(u1), Mux3/1
  Subsystem1/3(Desired LH Motor Torque) -> Subsystem4/2(u2), Mux3/2
  Subsystem3/1(Desired RK Motor Torque) -> Subsystem4/3(u3), Mux3/3
  Subsystem3/2(Desired LK Motor Torque) -> Subsystem4/4(u4), Mux3/4
  Subsystem4/1(Out1) -> Right Motor Torque Input/1
  Subsystem4/2(Out2) -> Right Motor Torque Input/2
  Subsystem4/3(Out3) -> Right Motor Torque Input/3
  Subsystem4/4(Out4) -> Left Motor Torque Input/1
  Subsystem4/5(Out5) -> Left Motor Torque Input/2
  Subsystem4/6(Out6) -> Left Motor Torque Input/3
  torqueFilter/1 -> Subsystem/11(alpha), Subsystem3/9(alpha), Subsystem1/1(alpha)
  Trigger/1 -> [Trigger]
  K p/1 -> Saturation/1, Mux/1
  K D/1 -> Saturation4/1, Mux/2
  Mux/1 -> K/1
  Saturation/1 -> Subsystem1/9(Kp Input), Subsystem3/7(Kp Input), Subsystem/7(Kp Input)
  Saturation4/1 -> Subsystem/8(KD Input), Subsystem1/10(KD Input), Subsystem3/8(KD Input)
  Subsystem7/1(RHA Desired) -> RHA Desired/1, [RHDA], Cast6/1
  Subsystem7/2(RKA Desired) -> RKA Desired/1, [RKDA], Cast4/1
  Subsystem7/4(LHA Desired) -> LHA Desired/1, [LHDA], Cast2/1
  Subsystem7/5(LKA Desired) -> [LKDA], Cast1/1, LKA Desired/1
  Subsystem7/6(LAA Desired) -> LAA Desired/1, [LADA], Cast5/1
  Fourier Series/2(Right_Knee_Desired) -> RKA Initial/1, Subsystem7/2(RKDA)
  Fourier Series/5(Left_Knee_Desired) -> LKA Initial/1, Subsystem7/5(LKDA)
  Fourier Series/4(Left_Hip_Desired) -> LHA Initial/1, Subsystem7/4(LHDA)
  Fourier Series/1(Right_Hip_Desired) -> RHA Initial/1, Subsystem7/1(RHDA)
  Fourier Series/6(Left_Ankle_Desired) -> LAA Initial/1, Subsystem7/6(LADA)
  Fourier Series/3(Right_Ankle_Desired) -> RAA Initial/1, Subsystem7/3(RADA)
  Cast5/1 -> Packet Output2/6
  Cast1/1 -> Packet Output2/5
  Cast2/1 -> Packet Output2/4
  Cast3/1 -> Packet Output2/3
  Cast4/1 -> Packet Output2/2
  Cast6/1 -> Packet Output2/1
  Subsystem7/9(LA Strategy) -> Left Strategy/1
  Subsystem7/8(RA Strategy) -> Right Strategy/1
  Subsystem7/7(Hip Strategy) -> Hip Strategy/1
  Subsystem7/3(RAA Desired) -> RAA Desired/1, [RADA], Cast3/1
  From1/1 -> Subsystem/1(A), Subsystem3/1(A), Subsystem1/2(A)
  [W] -> Subsystem3/2(W), Subsystem/2(W), Subsystem1/3(W)
  [hipOffset] -> Subsystem1/4(Offset)
  [W] -> If/1, Subsystem2/1(Input11)
  If/1 -> Subsystem2/Action
  [RHDA] -> Subsystem2/2(Right_Hip_Desired)
  [RKDA] -> Subsystem2/3(Right_Knee_Desired)
  [RADA] -> Subsystem2/4(Right_Ankle_Desired)
  [LHDA] -> Subsystem2/5(Left_Hip_Desired)
  [LKDA] -> Subsystem2/6(Left_Knee_Desired)
  gamma/1 -> Subsystem2/7(gamma)
  [LADA] -> Subsystem2/8(Left_Ankle_Desired)
  RKAA/1 -> [RKAA], Subsystem2/10(RKAA)
  RAAA/1 -> [RAAA], Subsystem2/11(RAAA)
  LHAA/1 -> [LHAA], Subsystem2/12(LHAA)
  LKAA/1 -> [LKAA], Subsystem2/13(LKAA)
  P_t_ZMP_Gain_hip/1 -> Subsystem2/14(P_t_ZMP_Gain_hip)
  LAAA/1 -> [LAAA], Subsystem2/15(LAAA)
  RHP/1 -> Pressure filtering/1(u)
  RTP/1 -> Pressure filtering/2(u1)
  LHP/1 -> Pressure filtering/3(u2)
  LTP/1 -> Pressure filtering/4(u3)
  ankleStrategyInterval/1 -> Subsystem2/20(ankleStrategyInterval)
  P_t_ZMP_Gain_Ankle/1 -> Subsystem2/21(P_t_ZMP_Gain_Ankle)
  m2/1 -> Subsystem2/22(m2)
  m3/1 -> Subsystem2/23(m3)
  m4/1 -> Subsystem2/24(m4)
  l_c2/1 -> Subsystem2/25(l_c2)
  l_c3/1 -> Subsystem2/26(l_c3)
  l_c4/1 -> Subsystem2/27(l_c4)
  I1/1 -> Subsystem2/28(I1)
  I2/1 -> Subsystem2/29(I2)
  I3/1 -> Subsystem2/30(I3)
  l3/1 -> Subsystem2/31(l3)
  l4/1 -> Subsystem2/32(l4)
  Subsystem2/6(currentStep/Time) -> currentStep/Time/1
  Subsystem2/7(Out11) -> Ankle Strategy/1
  Pressure filtering/2(y1) -> Subsystem2/17(RTP), [RTP]
  Pressure filtering/1(y) -> [RHP], Subsystem2/16(RHP)
  Pressure filtering/3(y2) -> [LHP], Subsystem2/18(LHP)
  Pressure filtering/4(y3) -> [LTP], Subsystem2/19(LTP)
  [RHP] -> Subsystem7/17(RHP)
  [LTP] -> Subsystem7/20(LTP)
  [LHP] -> Subsystem7/19(LHP)
  [RTP] -> Subsystem7/18(RTP)
  RHAA/1 -> [RHAA], Subsystem2/9(RHAA)
  [RHAA] -> Subsystem7/7(RHAA)
  [RKAA] -> Subsystem7/8(RKAA)
  [RAAA] -> Subsystem7/9(RAAA)
  [LHAA] -> Subsystem7/10(LHAA)
  [LKAA] -> Subsystem7/11(LKAA)
  [LAAA] -> Subsystem7/12(LAAA)
  Subsystem2/5(DCM Error) -> [DCMError], Scope/1
  [DCMError] -> Mux3/7
  Subsystem2/1(Out5) -> [RHS]
  [RHS] -> Subsystem7/13(RHS)
  Subsystem2/2(Out6) -> [LHS]
  [LHS] -> Subsystem7/14(LHS)
  Subsystem2/3(Out7) -> [RAS]
  Subsystem2/4(Out8) -> [LAS]
  [LAS] -> Subsystem7/15(LAS)
  [RAS] -> Subsystem7/16(RAS)
  [RHAA] -> Subsystem1/5(Right Hip Actual)
  [LHAA] -> Subsystem1/6(Left Hip Actual)
  [RHS] -> Subsystem1/11(Right Strategy)
  [LHS] -> Subsystem1/12(Left Strategy)
  [RKAA] -> Subsystem3/3(Right Knee Actual)
  [LKAA] -> Subsystem3/4(Left Knee Actual)
  [LAS] -> Subsystem/10(Left Strategy)
  [RAS] -> Subsystem/9(Right Strategy)
  [RAAA] -> Subsystem/3(Right Ankle Actual)
  [LAAA] -> Subsystem/4(Left Ankle Actual)
  Subsystem7/10(Strategy Gain) -> Product3/2
  Product3/1 -> Scope2/1, Strategy Gain/1
  [Gain] -> Product3/1
  Subsystem2/8(Out1) -> Scope1/1, [Gain]
  [Trigger] -> Subsystem7/21(Trigger)
  [Trigger] -> Subsystem4/7(Trigger)

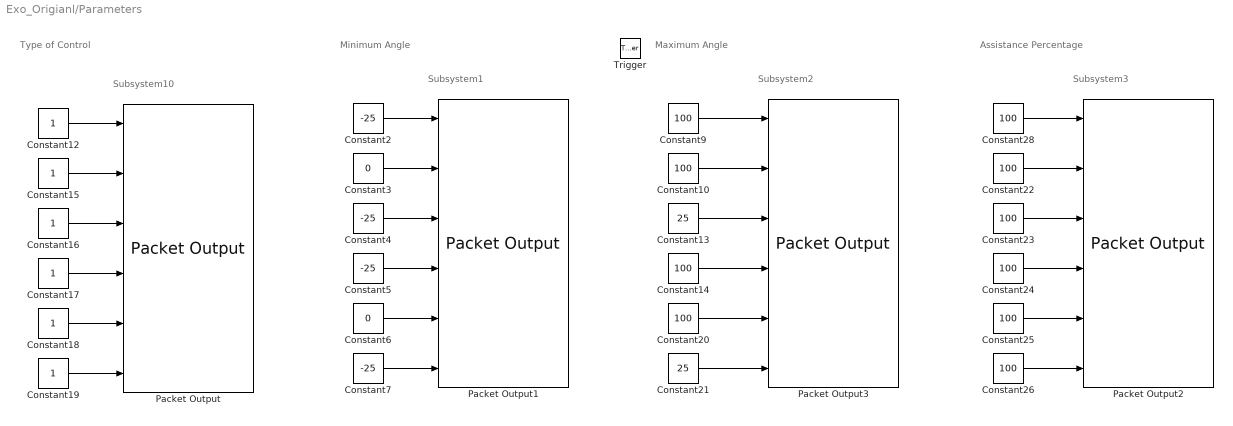
== system Exo_Origianl/Parameters ==
  note: Subsystem2
  note: Subsystem3
  note: Subsystem1
  note: Subsystem10
  note: Minimum Angle
  note: Assistance Percentage
  note: Type of Control
  note: Maximum Angle
  Trigger : TriggerPort  VariantControl=(inherit)  PortDimensions=1
  Constant{9..10,14,20,22..26,28} (10 alike) : Constant  Value=100
  Constant{12,15..19} (6 alike) : Constant
  Constant13 : Constant  Value=25
  Constant{2,4..5,7} (4 alike) : Constant  Value=-25
  Constant21 : Constant  Value=25
  Constant3 : Constant  Value=0
  Constant6 : Constant  Value=0
  Packet Output : sldrtlib/Packet Output  SampleTime=-1  MaxMissedTicks=100  ShowMissedTicks=off  YieldWhenWaiting=off  DrvName=PEAK-System/CAN_Device  DrvAddress=81  DrvOptions=[0 0 0 0 1000 0 0 1 5 2 1 3 1]  PacketSize=6  DataTypes={'uint8','uint8','uint8','uint8','uint8','uint8'}  ShowReady=off  ShowError=off  PacketID=2048e0 + (71)  ByteOrder=2  InitialValue=[]  FinalValue=[]
      settings: AttributesFormatString=PEAK-System\nCAN Device [81]
  Packet Output1 : sldrtlib/Packet Output  SampleTime=-1  MaxMissedTicks=100  ShowMissedTicks=off  YieldWhenWaiting=off  DrvName=PEAK-System/CAN_Device  DrvAddress=81  DrvOptions=[0 0 0 0 1000 0 0 1 5 2 1 3 1]  PacketSize=6  DataTypes={'int8','int8','int8','int8','int8','int8'}  ShowReady=off  ShowError=off  PacketID=2048e0 + (75)  ByteOrder=2  InitialValue=[]  FinalValue=[]
      settings: AttributesFormatString=PEAK-System\nCAN Device [81]
  Packet Output2 : sldrtlib/Packet Output  SampleTime=-1  MaxMissedTicks=100  ShowMissedTicks=off  YieldWhenWaiting=off  DrvName=PEAK-System/CAN_Device  DrvAddress=81  DrvOptions=[0 0 0 0 1000 0 0 1 5 2 1 3 1]  PacketSize=6  DataTypes={'int8','int8','int8','int8','int8','int8'}  ShowReady=off  ShowError=off  PacketID=2048e0 + (76)  ByteOrder=2  InitialValue=[]  FinalValue=[]
      settings: AttributesFormatString=PEAK-System\nCAN Device [81]
  Packet Output3 : sldrtlib/Packet Output  SampleTime=-1  MaxMissedTicks=100  ShowMissedTicks=off  YieldWhenWaiting=off  DrvName=PEAK-System/CAN_Device  DrvAddress=81  DrvOptions=[0 0 0 0 1000 0 0 1 5 2 1 3 1]  PacketSize=6  DataTypes={'int8','int8','int8','int8','int8','int8'}  ShowReady=off  ShowError=off  PacketID=2048e0 + (80)  ByteOrder=2  InitialValue=[]  FinalValue=[]
      settings: AttributesFormatString=PEAK-System\nCAN Device [81]
  wires:
  Constant17/1 -> Packet Output/4
  Constant18/1 -> Packet Output/5
  Constant19/1 -> Packet Output/6
  Constant12/1 -> Packet Output/1
  Constant15/1 -> Packet Output/2
  Constant16/1 -> Packet Output/3
  Constant5/1 -> Packet Output1/4
  Constant6/1 -> Packet Output1/5
  Constant7/1 -> Packet Output1/6
  Constant2/1 -> Packet Output1/1
  Constant3/1 -> Packet Output1/2
  Constant4/1 -> Packet Output1/3
  Constant24/1 -> Packet Output2/4
  Constant25/1 -> Packet Output2/5
  Constant26/1 -> Packet Output2/6
  Constant28/1 -> Packet Output2/1
  Constant22/1 -> Packet Output2/2
  Constant23/1 -> Packet Output2/3
  Constant14/1 -> Packet Output3/4
  Constant20/1 -> Packet Output3/5
  Constant21/1 -> Packet Output3/6
  Constant9/1 -> Packet Output3/1
  Constant10/1 -> Packet Output3/2
  Constant13/1 -> Packet Output3/3

== system Exo_Origianl/Read Angular Possition ==
  Input : Inport
  If : If  IfExpression=u1 == 1
  If Action Subsystem : Subsystem  TreatAsAtomicUnit=on
  If Action Subsystem1 : Subsystem  TreatAsAtomicUnit=on
  Merge{,1..5} (6 alike) : Merge
  Out1 : Outport
  Out2 : Outport  Port=2
  Out3 : Outport  Port=3
  Out4 : Outport  Port=4
  Out5 : Outport  Port=5
  Out6 : Outport  Port=6
  wires:
  Input/1 -> If/1
  Merge/1 -> Out1/1
  If Action Subsystem/1(Out7) -> Merge/1
  If/1 -> If Action Subsystem/Action
  If/2 -> If Action Subsystem1/Action
  Merge1/1 -> Out2/1
  Merge2/1 -> Out3/1
  Merge3/1 -> Out4/1
  Merge4/1 -> Out5/1
  Merge5/1 -> Out6/1
  If Action Subsystem/2(Out8) -> Merge1/1
  If Action Subsystem/3(Out9) -> Merge2/1
  If Action Subsystem/4(Out10) -> Merge3/1
  If Action Subsystem/5(Out11) -> Merge4/1
  If Action Subsystem/6(Out12) -> Merge5/1
  If Action Subsystem1/1(Out7) -> Merge/2
  If Action Subsystem1/2(Out8) -> Merge1/2
  If Action Subsystem1/3(Out9) -> Merge2/2
  If Action Subsystem1/4(Out10) -> Merge3/2
  If Action Subsystem1/5(Out11) -> Merge4/2
  If Action Subsystem1/6(Out12) -> Merge5/2

== system Exo_Origianl/Read Angular Velocity ==
  Input : Inport
  If : If  IfExpression=u1 == 1
  If Action Subsystem1 : Subsystem  TreatAsAtomicUnit=on
  Out1 : Outport
  Out2 : Outport  Port=2
  Out3 : Outport  Port=3
  Out4 : Outport  Port=4
  Out5 : Outport  Port=5
  Out6 : Outport  Port=6
  wires:
  Input/1 -> If/1
  If/2 -> If Action Subsystem1/Action
  If Action Subsystem1/1(Out7) -> Out1/1
  If Action Subsystem1/2(Out8) -> Out2/1
  If Action Subsystem1/3(Out9) -> Out3/1
  If Action Subsystem1/4(Out10) -> Out4/1
  If Action Subsystem1/5(Out11) -> Out5/1
  If Action Subsystem1/6(Out12) -> Out6/1

== system Exo_Origianl/Read Interaction torque ==
  Input : Inport
  If : If  IfExpression=u1 == 1
  If Action Subsystem : Subsystem  TreatAsAtomicUnit=on
  If Action Subsystem1 : Subsystem  TreatAsAtomicUnit=on
  Merge{,1..5} (6 alike) : Merge
  Out1 : Outport
  Out2 : Outport  Port=2
  Out3 : Outport  Port=3
  Out4 : Outport  Port=4
  Out5 : Outport  Port=5
  Out6 : Outport  Port=6
  wires:
  Input/1 -> If/1
  Merge/1 -> Out1/1
  If Action Subsystem/1(Out7) -> Merge/1
  If/1 -> If Action Subsystem/Action
  If/2 -> If Action Subsystem1/Action
  Merge1/1 -> Out2/1
  Merge2/1 -> Out3/1
  Merge3/1 -> Out4/1
  Merge4/1 -> Out5/1
  Merge5/1 -> Out6/1
  If Action Subsystem/2(Out8) -> Merge1/1
  If Action Subsystem/3(Out9) -> Merge2/1
  If Action Subsystem/4(Out10) -> Merge3/1
  If Action Subsystem/5(Out11) -> Merge4/1
  If Action Subsystem/6(Out12) -> Merge5/1
  If Action Subsystem1/1(Out7) -> Merge/2
  If Action Subsystem1/2(Out8) -> Merge1/2
  If Action Subsystem1/3(Out9) -> Merge2/2
  If Action Subsystem1/4(Out10) -> Merge3/2
  If Action Subsystem1/5(Out11) -> Merge4/2
  If Action Subsystem1/6(Out12) -> Merge5/2

== system Exo_Origianl/Read Motor torque ==
  Input : Inport
  If : If  IfExpression=u1 == 1
  If Action Subsystem : Subsystem  TreatAsAtomicUnit=on
  If Action Subsystem1 : Subsystem  TreatAsAtomicUnit=on
  Merge{,1..5} (6 alike) : Merge
  Out1 : Outport
  Out2 : Outport  Port=2
  Out3 : Outport  Port=3
  Out4 : Outport  Port=4
  Out5 : Outport  Port=5
  Out6 : Outport  Port=6
  wires:
  Input/1 -> If/1
  Merge/1 -> Out1/1
  If Action Subsystem/1(Out7) -> Merge/1
  If/1 -> If Action Subsystem/Action
  If/2 -> If Action Subsystem1/Action
  Merge1/1 -> Out2/1
  Merge2/1 -> Out3/1
  Merge3/1 -> Out4/1
  Merge4/1 -> Out5/1
  Merge5/1 -> Out6/1
  If Action Subsystem/2(Out8) -> Merge1/1
  If Action Subsystem/3(Out9) -> Merge2/1
  If Action Subsystem/4(Out10) -> Merge3/1
  If Action Subsystem/5(Out11) -> Merge4/1
  If Action Subsystem/6(Out12) -> Merge5/1
  If Action Subsystem1/1(Out7) -> Merge/2
  If Action Subsystem1/2(Out8) -> Merge1/2
  If Action Subsystem1/3(Out9) -> Merge2/2
  If Action Subsystem1/4(Out10) -> Merge3/2
  If Action Subsystem1/5(Out11) -> Merge4/2
  If Action Subsystem1/6(Out12) -> Merge5/2

== system Exo_Origianl/Subsystem ==
  In1 : Inport
  In2 : Inport  Port=2
  Trigger : TriggerPort  VariantControl=(inherit)  PortDimensions=1
  Constant{1..6} (6 alike) : Constant  Value=4
  Packet Output : sldrtlib/Packet Output  SampleTime=-1  MaxMissedTicks=100  ShowMissedTicks=off  YieldWhenWaiting=off  DrvName=PEAK-System/CAN_Device  DrvAddress=81  DrvOptions=[0 0 0 0 1000 0 0 1 5 2 1 3 1]  PacketSize=8  DataTypes={'uint8','uint8','uint8','uint8','uint8','uint8','uint8','uint8'}  ShowReady=off  ShowError=off  PacketID=2048e0 + (81)  ByteOrder=2  InitialValue=[]  FinalValue=[]
      settings: AttributesFormatString=PEAK-System\nCAN Device [81]
  wires:
  Constant3/1 -> Packet Output/4
  In1/1 -> Packet Output/1
  Constant5/1 -> Packet Output/6
  Constant4/1 -> Packet Output/5
  In2/1 -> Packet Output/2
  Constant2/1 -> Packet Output/3
  Constant1/1 -> Packet Output/7
  Constant6/1 -> Packet Output/8
